simulink model "planar5link"  (R2018b)
settings: Solver=ode4  StartTime=0.0  StopTime=12  FixedStep=0.001  RelTol=1e-3
libraries: simulink x1
settings Model: Creator=User  LastModifiedBy=User

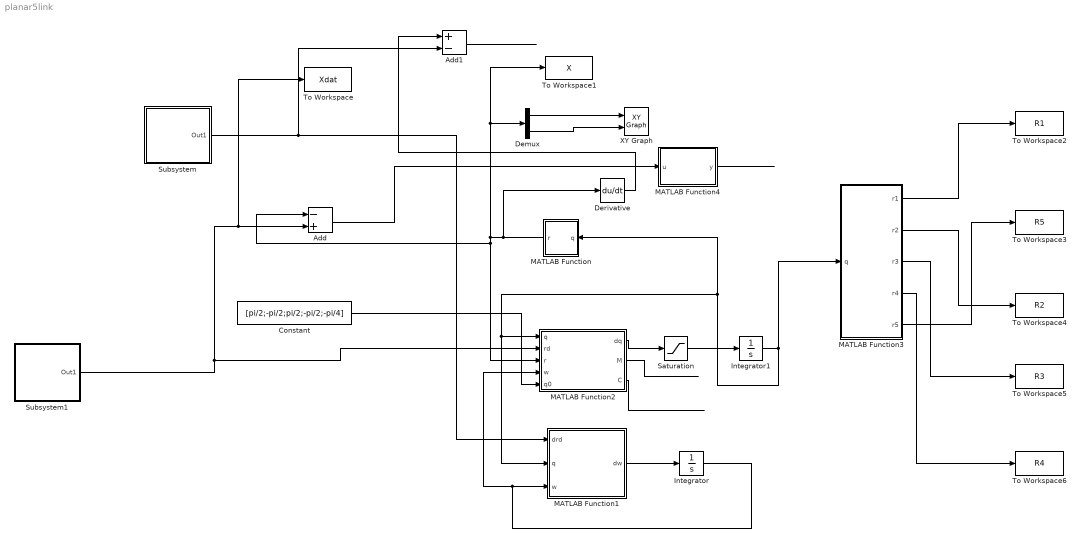
== system planar5link ==
  Add : Sum  Inputs=-+
  Add1 : Sum  Inputs=+-
  Constant : Constant  Value=[pi/2;-pi/2;pi/2;-pi/2;-pi/4]
  Demux : Demux  Outputs=2
  Derivative : Derivative
  Integrator : Integrator  InitialCondition=[0;0]
  Integrator1 : Integrator  InitialCondition=[pi/2;-pi/2;pi/2;-pi/2;-pi/4]
  MATLAB Function : MATLAB Function  TreatAsAtomicUnit=on
  MATLAB Function1 : MATLAB Function  TreatAsAtomicUnit=on
  MATLAB Function2 : MATLAB Function  TreatAsAtomicUnit=on
  MATLAB Function3 : MATLAB Function  TreatAsAtomicUnit=on
  MATLAB Function4 : MATLAB Function  TreatAsAtomicUnit=on
  Saturation : Saturate  UpperLimit=ones(5,1)*0.21  LowerLimit=-0.21*ones(5,1)
  Subsystem : Subsystem
  Subsystem1 : Subsystem
  To Workspace : ToWorkspace  VariableName=Xdat  SampleTime=-1
  To Workspace1 : ToWorkspace  VariableName=X  SampleTime=-1
  To Workspace2 : ToWorkspace  VariableName=R1  SampleTime=-1
  To Workspace3 : ToWorkspace  VariableName=R5  SampleTime=-1
  To Workspace4 : ToWorkspace  VariableName=R2  SampleTime=-1
  To Workspace5 : ToWorkspace  VariableName=R3  SampleTime=-1
  To Workspace6 : ToWorkspace  VariableName=R4  SampleTime=-1
  XY Graph : simulink/Sinks/XY Graph  xmin=1.5  xmax=3.5  ymin=1  ymax=2.5  st=-1
  wires:
  MATLAB Function1/1(dw) -> Integrator/1
  Integrator/1 -> MATLAB Function2/4(w), MATLAB Function1/3(w)
  Subsystem/1(Out1) -> Add1/2, MATLAB Function1/1(drd)
  MATLAB Function2/1(dq) -> Saturation/1
  Integrator1/1 -> MATLAB Function3/1(q), MATLAB Function1/2(q), MATLAB Function2/1(q), MATLAB Function/1(q)
  MATLAB Function/1(r) -> Add/1, MATLAB Function2/3(r), To Workspace1/1, Demux/1, Derivative/1
  Subsystem1/1(Out1) -> To Workspace/1, Add/2, MATLAB Function2/2(rd)
  Saturation/1 -> Integrator1/1
  Constant/1 -> MATLAB Function2/5(q0)
  Derivative/1 -> Add1/1
  Demux/1 -> XY Graph/1
  Demux/2 -> XY Graph/2
  Add/1 -> MATLAB Function4/1(u)
  MATLAB Function2/2(M) -> ?
  Add1/1 -> ?
  MATLAB Function3/1(r1) -> To Workspace2/1
  MATLAB Function3/2(r2) -> To Workspace4/1
  MATLAB Function3/3(r3) -> To Workspace5/1
  MATLAB Function3/4(r4) -> To Workspace6/1
  MATLAB Function3/5(r5) -> To Workspace3/1
  MATLAB Function4/1(y) -> ?
  MATLAB Function2/3(C) -> ?

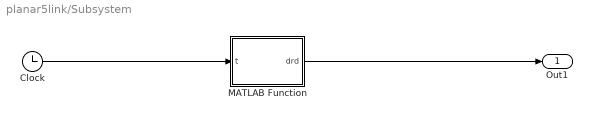
== system planar5link/Subsystem ==
  Clock : Clock
  MATLAB Function : MATLAB Function  TreatAsAtomicUnit=on
  Out1 : Outport
  wires:
  MATLAB Function/1(drd) -> Out1/1
  Clock/1 -> MATLAB Function/1(t)

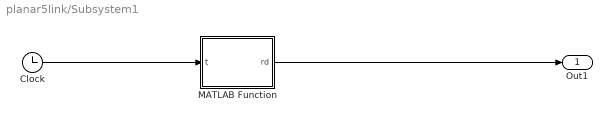
== system planar5link/Subsystem1 ==
  Clock : Clock
  MATLAB Function : MATLAB Function  TreatAsAtomicUnit=on
  Out1 : Outport
  wires:
  Clock/1 -> MATLAB Function/1(t)
  MATLAB Function/1(rd) -> Out1/1

== matlab function planar5link/Subsystem/MATLAB Function ==
  data: t input; drd output
function drd = fcn(t)
if (t>=0) && (t<=4)
    drd=[-0.05991*t^2+0.2397*t;
        -0.1038*t^2+0.4152*t];
elseif (t<=8)
    drd=[0.11985*(t-4)^2-0.4794*(t-4);
        0];
else 
    drd=[-0.05991*(t-8)^2+0.2397*(t-8);
        0.1038*(t-8)^2-0.4152*(t-8)];
end
end

== matlab function planar5link/MATLAB Function ==
  data: q input; r output
function r = fcn(q)
q1=q(1);
q2=q(2);
q3=q(3);
q4=q(4);
q5=q(5);
r=[cos(q1)+cos(q1+q2)+cos(q1+q2+q3)+cos(q1+q2+q3+q4)+cos(q1+q2+q3+q4+q5);
   sin(q1)+sin(q1+q2)+sin(q1+q2+q3)+sin(q1+q2+q3+q4)+sin(q1+q2+q3+q4+q5)];
end

== matlab function planar5link/MATLAB Function1 ==
  data: drd input; dw output; q input; w input
function dw = fcn(drd,q,w)
q1=q(1);
q2=q(2);
q3=q(3);
q4=q(4);
q5=q(5);
muy=0.02;
J=[-sin(q1)-sin(q1+q2)-sin(q1+q2+q3)-sin(q1+q2+q3+q4)-sin(q1+q2+q3+q4+q5) -sin(q1+q2)-sin(q1+q2+q3)-sin(q1+q2+q3+q4)-sin(q1+q2+q3+q4+q5) -sin(q1+q2+q3)-sin(q1+q2+q3+q4)-sin(q1+q2+q3+q4+q5) -sin(q1+q2+q3+q4)-sin(q1+q2+q3+q4+q5) -sin(q1+q2+q3+q4+q5);
    cos(q1)+cos(q1+q2)+cos(q1+q2+q3)+cos(q1+q2+q3+q4)+cos(q1+q2+q3+q4+q5) cos(q1+q2)+cos(q1+q2+q3)+cos(q1+q2+q3+q4)+cos(q1+q2+q3+q4+q5) cos(q1+q2+q3)+cos(q1+q2+q3+q4)+cos(q1+q2+q3+q4+q5) cos(q1+q2+q3+q4)+cos(q1+q2+q3+q4+q5) cos(q1+q2+q3+q4+q5)];
dw=(drd-J*J'*w)/muy;
end

== matlab function planar5link/MATLAB Function2 ==
  data: q input; dq output; rd input; r input; w input; M output; q0 input; C output
function [dq,M,C] = fcn(q,rd,r,w,q0)
q1=q(1);
q2=q(2);
q3=q(3);
q4=q(4);
q5=q(5);
gamma=100;
kappa=0.42;
J=[-sin(q1)-sin(q1+q2)-sin(q1+q2+q3)-sin(q1+q2+q3+q4)-sin(q1+q2+q3+q4+q5) -sin(q1+q2)-sin(q1+q2+q3)-sin(q1+q2+q3+q4)-sin(q1+q2+q3+q4+q5) -sin(q1+q2+q3)-sin(q1+q2+q3+q4)-sin(q1+q2+q3+q4+q5) -sin(q1+q2+q3+q4)-sin(q1+q2+q3+q4+q5) -sin(q1+q2+q3+q4+q5);
    cos(q1)+cos(q1+q2)+cos(q1+q2+q3)+cos(q1+q2+q3+q4)+cos(q1+q2+q3+q4+q5) cos(q1+q2)+cos(q1+q2+q3)+cos(q1+q2+q3+q4)+cos(q1+q2+q3+q4+q5) cos(q1+q2+q3)+cos(q1+q2+q3+q4)+cos(q1+q2+q3+q4+q5) cos(q1+q2+q3+q4)+cos(q1+q2+q3+q4+q5) cos(q1+q2+q3+q4+q5)];
dq=gamma*J'*(rd-r)+J'*w-kappa*(q-q0);
M=min(eig(J*J'));
C=pinv(J')*(q-q0);
end

== matlab function planar5link/Subsystem1/MATLAB Function ==
  data: t input; rd output
function rd  = fcn(t)
if (t>=0) && (t<=4)
    rd=[-0.01997*t^3+0.11985*t^2+2+cosd(45);
        -0.0346*t^3+0.2076*t^2+2-cosd(45)];
elseif (t<=8)
    rd=[0.03995*(t-4)^3-0.2397*(t-4)^2+2+cosd(45)+(0.4+cosd(45))/sqrt(3);
        2.4];
else 
    rd=[-0.01997*(t-8)^3+0.11985*(t-8)^2+2+cosd(45)-(0.4+cosd(45))/sqrt(3);
        0.0346*(t-8)^3-0.2076*(t-8)^2+2.4];
end
% q1=pi/2;
% q2=-pi/2;
% q3=pi/2;
% x=rd(1);
% y=rd(2);
% r=sqrt((x-1)^2+(y-2)^2);
% q5=2*acos(r/2)-pi;
% phi=atan2(y-2,x-1);
% q4=phi+acos(r/2)-pi/2;
% q0=[q1;q2;q3;q4;q5];
end

== matlab function planar5link/MATLAB Function3 ==
  data: q input; r1 output; r2 output; r3 output; r4 output; r5 output
function [r1,r2,r3,r4,r5] = fcn(q)
q1=q(1);
q2=q(2);
q3=q(3);
q4=q(4);
q5=q(5);
r5=[cos(q1)+cos(q1+q2)+cos(q1+q2+q3)+cos(q1+q2+q3+q4)+cos(q1+q2+q3+q4+q5);
   sin(q1)+sin(q1+q2)+sin(q1+q2+q3)+sin(q1+q2+q3+q4)+sin(q1+q2+q3+q4+q5)];
r4=[cos(q1)+cos(q1+q2)+cos(q1+q2+q3)+cos(q1+q2+q3+q4);
   sin(q1)+sin(q1+q2)+sin(q1+q2+q3)+sin(q1+q2+q3+q4)];
r3=[cos(q1)+cos(q1+q2)+cos(q1+q2+q3);
   sin(q1)+sin(q1+q2)+sin(q1+q2+q3)];
r2=[cos(q1)+cos(q1+q2);
   sin(q1)+sin(q1+q2)];
r1=[cos(q1);
   sin(q1)];
end

== matlab function planar5link/MATLAB Function4 ==
  data: u input; y output
function y = fcn(u)
y=norm(u,2);
end
